simulink model "HDLRxHeader"  (R2024a)
settings: Solver=VariableStepAuto  StartTime=0.0  StopTime=stopTime  RelTol=1e-3
undefined symbols (not defined in the file or in its folder): fPHY
libraries: dspsrcs4 x2, HDL_ieee_8021513 x2
settings Model: Creator=cotti  LastModifiedBy=cotti

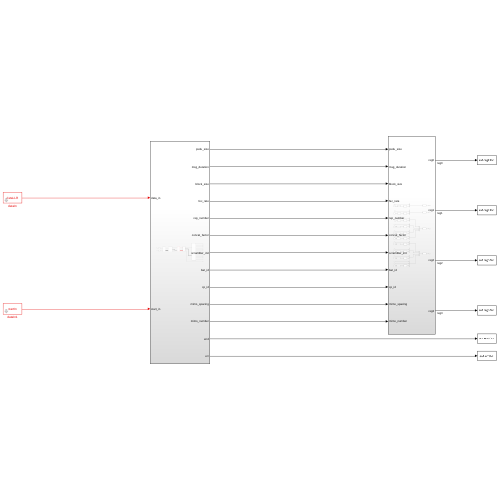
[thumbnail: Simulink's stored preview of the top-level diagram]
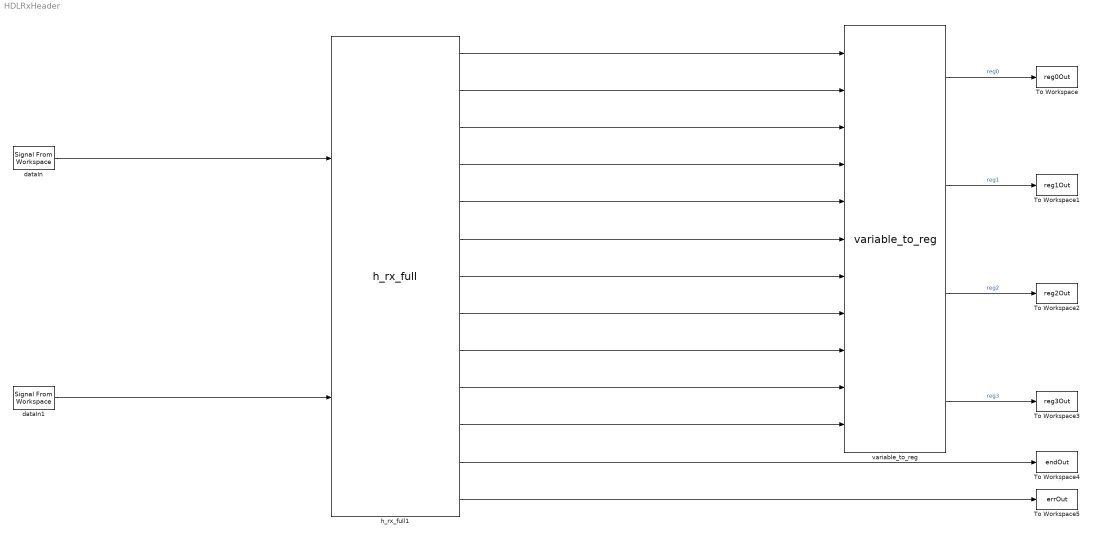
== system HDLRxHeader ==
  To Workspace : ToWorkspace  VariableName=reg0Out  SampleTime=4/fPHY
      settings: Save2DSignal=2-D array (concatenate along first dimension)
  To Workspace1 : ToWorkspace  VariableName=reg1Out  SampleTime=4/fPHY
      settings: Save2DSignal=2-D array (concatenate along first dimension)
  To Workspace2 : ToWorkspace  VariableName=reg2Out  SampleTime=4/fPHY
      settings: Save2DSignal=2-D array (concatenate along first dimension)
  To Workspace3 : ToWorkspace  VariableName=reg3Out  SampleTime=4/fPHY
      settings: Save2DSignal=2-D array (concatenate along first dimension)
  To Workspace4 : ToWorkspace  VariableName=endOut  SampleTime=4/fPHY
      settings: Save2DSignal=2-D array (concatenate along first dimension)
  To Workspace5 : ToWorkspace  VariableName=errOut  SampleTime=4/fPHY
      settings: Save2DSignal=2-D array (concatenate along first dimension)
  dataIn : dspsrcs4/Signal From Workspace  X=dataLLR  Ts=1/(2*fPHY)  nsamps=1  OutputAfterFinalValue=Setting to zero  ignoreOrWarnInputAndFrameLengths=off  OutputFrames=off
  dataIn1 : dspsrcs4/Signal From Workspace  X=startIn  Ts=1/(2*fPHY)  nsamps=1  OutputAfterFinalValue=Setting to zero  ignoreOrWarnInputAndFrameLengths=off  OutputFrames=off
  h_rx_full1 : HDL_ieee_8021513/h_rx_full  SystemSampleTime=-1  VariantActivationTime=update diagram  AllowFlexibleInterface=on  Latency=0  AutoFrameSizeCalculation=off
      settings: SourceProductName=HDL IEEE 8021513
  variable_to_reg : HDL_ieee_8021513/variable_to_reg  SystemSampleTime=-1  VariantActivationTime=update diagram  AllowFlexibleInterface=on  Latency=0  AutoFrameSizeCalculation=off
      settings: SourceProductName=HDL IEEE 8021513
  wires:
  h_rx_full1/1 -> variable_to_reg/1
  h_rx_full1/2 -> variable_to_reg/2
  h_rx_full1/3 -> variable_to_reg/3
  h_rx_full1/4 -> variable_to_reg/4
  h_rx_full1/5 -> variable_to_reg/5
  h_rx_full1/6 -> variable_to_reg/6
  h_rx_full1/7 -> variable_to_reg/7
  h_rx_full1/8 -> variable_to_reg/8
  h_rx_full1/9 -> variable_to_reg/9
  h_rx_full1/10 -> variable_to_reg/10
  h_rx_full1/11 -> variable_to_reg/11
  variable_to_reg/1 -> To Workspace/1  "reg0"
  variable_to_reg/2 -> To Workspace1/1  "reg1"
  variable_to_reg/3 -> To Workspace2/1  "reg2"
  variable_to_reg/4 -> To Workspace3/1  "reg3"
  h_rx_full1/12 -> To Workspace4/1
  h_rx_full1/13 -> To Workspace5/1
  dataIn/1 -> h_rx_full1/1
  dataIn1/1 -> h_rx_full1/2
